simulink model "w2p4"  (R2020b)
settings: Solver=VariableStepAuto  StartTime=0.0  StopTime=10.0  RelTol=1e-3
undefined symbols (not defined in the file): b, J, Ke, Kt, L, R
settings Model: Creator=k.Raviteja  LastModifiedBy=k.Raviteja

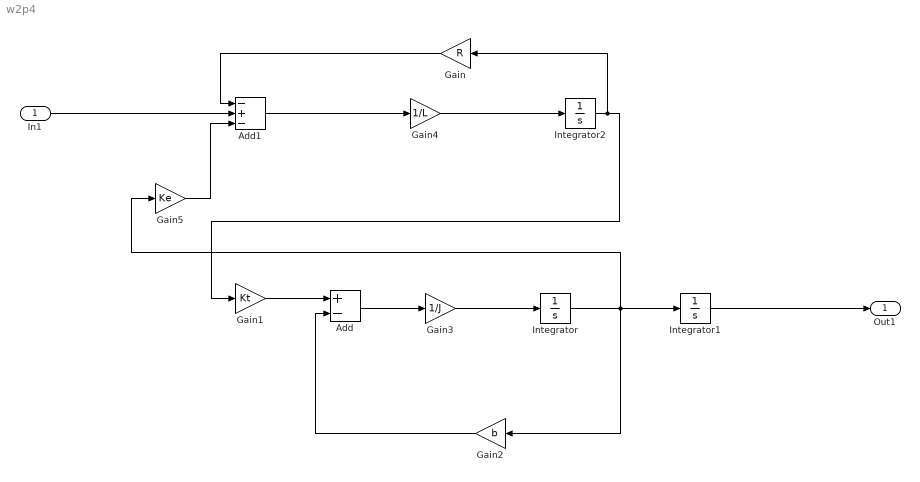
== system w2p4 ==
  In1 : Inport
  Add : Sum  Inputs=+-
  Add1 : Sum  Inputs=-+-
  Gain : Gain  Gain=R
  Gain1 : Gain  Gain=Kt
  Gain2 : Gain  Gain=b
  Gain3 : Gain  Gain=1/J
  Gain4 : Gain  Gain=1/L
  Gain5 : Gain  Gain=Ke
  Integrator : Integrator
  Integrator1 : Integrator
  Integrator2 : Integrator
  Out1 : Outport
  wires:
  Integrator/1 -> Gain5/1, Gain2/1, Integrator1/1
  Add1/1 -> Gain4/1
  Gain4/1 -> Integrator2/1
  Gain1/1 -> Add/1
  Gain3/1 -> Integrator/1
  Add/1 -> Gain3/1
  Integrator1/1 -> Out1/1
  Gain2/1 -> Add/2
  Integrator2/1 -> Gain/1, Gain1/1
  Gain5/1 -> Add1/3
  Gain/1 -> Add1/1
  In1/1 -> Add1/2
